simulink model "simLQR"  (R2015a)
settings: Solver=ode4  StartTime=0.0  StopTime=120  FixedStep=T  RelTol=1e-3
values from neighbouring files (symbols this model uses):
  aLeq = pnt(4)    [Data.m]
  aReq = pnt(3)    [Data.m]
  InitialValue = [0;0;0;rolleq;pitcheq;0;aReq;aLeq;0;0;0;0;0;0;0;0;reshape(AUX,256,1)]    [LinearAnalisys.m]
  pitcheq = pnt(2)    [Data.m]
  rolleq = pnt(1)    [Data.m]
  T = 12*(10^(-3))    (= 0.012)    [LinearAnalisys.m]
undefined symbols (not defined in the file or in its folder): K
settings Model: Creator=arthur  LastModifiedBy=macro
settings DebuggingCC: UnderspecifiedInitializationDetection=Classic  MergeDetectMultiDrivingBlocksExec=none  SolverPrmCheckMsg=warning  StateNameClashWarn=warning

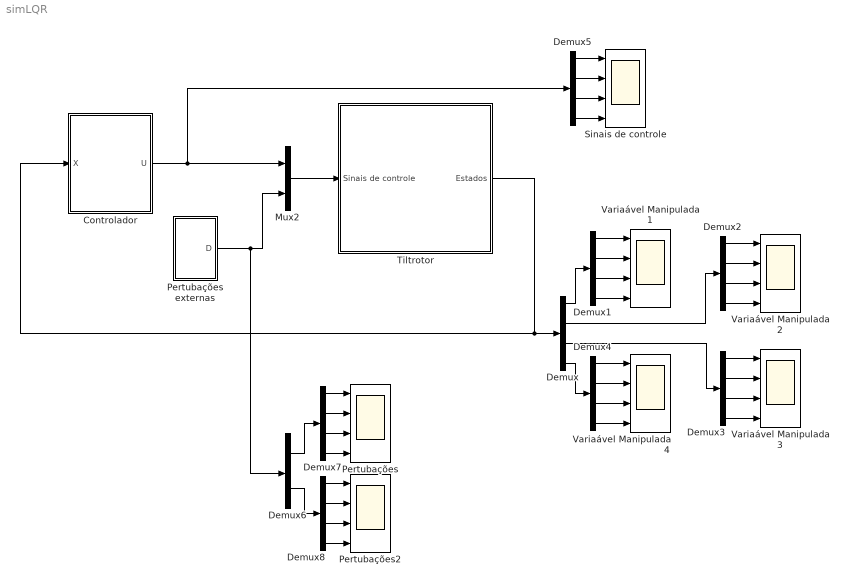
== system simLQR ==
  Controlador : Subsystem
      mask Display: image(imread('Photos/pc.jpg'))
  Demux{,1..5,7..8} (8 alike) : Demux
  Demux6 : Demux  Outputs=2
  Mux2 : Mux  Inputs=[4,8]
  Pertubações : Scope  NumInputPorts=4
      settings: YMin=-0.035~-0.5~-0.03~-0.3  YMax=0.005~3~0.005~0.05
  Pertubações externas : Subsystem
  Pertubações2 : Scope  NumInputPorts=4
      settings: YMin=-0.035~-0.5~-0.03~-0.3  YMax=0.005~3~0.005~0.05  SaveName=ScopeData2
  Sinais de controle : Scope  NumInputPorts=4
      settings: YMin=-0.035~-0.5~-0.03~-0.3  YMax=0.005~3~0.005~0.05
  Tiltrotor : Subsystem
      mask Display: image(imread('Photos/tilt.jpg'))
  Variaável Manipulada{1..4} (4 alike) : Scope  NumInputPorts=4
      Variaável Manipulada1 settings: YMin=-0.02~0.001~-0.08~0  YMax=0.05~0.009~-0.01~7  SaveName=ScopeData3
      Variaável Manipulada2 settings: YMin=-2~-55~-4250~-4000  YMax=2~-20~-2250~-2250  SaveName=ScopeData6
      Variaável Manipulada3 settings: YMin=-0.0045~-5~-5~-5  YMax=0.002~5~5~5  SaveName=ScopeData4
      Variaável Manipulada4 settings: YMin=0.055~-0.0195~-0.06475~-0.11  YMax=0.058~-0.0165~-0.06325~-0.055  SaveName=ScopeData5
  wires:
  Mux2/1 -> Tiltrotor/1(Sinais de controle)
  Pertubações externas/1(D) -> Demux6/1, Mux2/2
  Tiltrotor/1(Estados) -> Demux/1, Controlador/1(X)
  Demux/1 -> Demux1/1
  Demux1/1 -> Variaável Manipulada1/1
  Demux1/2 -> Variaável Manipulada1/2
  Demux1/3 -> Variaável Manipulada1/3
  Demux1/4 -> Variaável Manipulada1/4
  Demux/2 -> Demux2/1
  Demux2/1 -> Variaável Manipulada2/1
  Demux2/2 -> Variaável Manipulada2/2
  Demux2/3 -> Variaável Manipulada2/3
  Demux2/4 -> Variaável Manipulada2/4
  Demux/3 -> Demux3/1
  Demux3/1 -> Variaável Manipulada3/1
  Demux3/2 -> Variaável Manipulada3/2
  Demux3/3 -> Variaável Manipulada3/3
  Demux3/4 -> Variaável Manipulada3/4
  Demux/4 -> Demux4/1
  Demux4/1 -> Variaável Manipulada4/1
  Demux4/2 -> Variaável Manipulada4/2
  Demux4/3 -> Variaável Manipulada4/3
  Demux4/4 -> Variaável Manipulada4/4
  Demux5/1 -> Sinais de controle/1
  Demux5/2 -> Sinais de controle/2
  Demux5/3 -> Sinais de controle/3
  Demux5/4 -> Sinais de controle/4
  Demux6/1 -> Demux7/1
  Demux7/1 -> Pertubações/1
  Demux7/2 -> Pertubações/2
  Demux7/3 -> Pertubações/3
  Demux7/4 -> Pertubações/4
  Demux6/2 -> Demux8/1
  Demux8/1 -> Pertubações2/1
  Demux8/2 -> Pertubações2/2
  Demux8/3 -> Pertubações2/3
  Demux8/4 -> Pertubações2/4
  Controlador/1(U) -> Mux2/1, Demux5/1

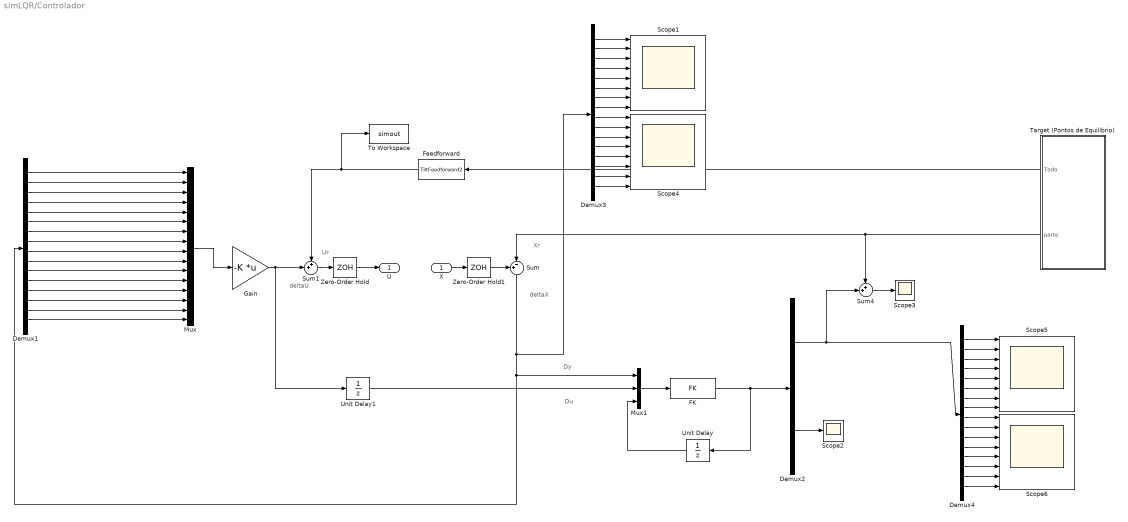
== system simLQR/Controlador ==
  note: Du
  note: Dy
  note: Xr
  note: deltaX
  note: Ur
  note: deltaU
  X : Inport
  Demux1 : Demux  Outputs=16
  Demux2 : Demux  Outputs=[16,256]
  Demux3 : Demux  Outputs=16
  Demux4 : Demux  Outputs=16
  FK : MATLABFcn  MATLABFcn=FK  OutputDimensions=272
  Feedforward : MATLABFcn  MATLABFcn=TiltFeedforward2  OutputDimensions=4
  Gain : Gain  Gain=-K  Multiplication=Matrix(K*u) (u vector)
  Mux : Mux  Inputs=16
  Mux1 : Mux  Inputs=[16,4,272]
  Scope{1,4..6} (4 alike) : Scope  NumInputPorts=8
      Scope1 settings: YMin=-0.0001~-0.000125~-0.00015~0.001925~0.052~0.0005~-0.05466~-0.05164  YMax=0.0009~2.5e-05~5e-05~0.002075~0.05375~0.0035~-0.05461~-0.05159  SaveName=ScopeData8
      Scope4 settings: YMin=-0.055~-5~-5~-5~-5~-5~-5~-5  YMax=0.055~5~5~5~5~5~5~5  SaveName=ScopeData11
      Scope5 settings: YMin=0.00075~7.5e-05~-9e-05~-0.00749~0.0434~0.00125~-0.04485~-0.042475  YMax=0.002~0.0002~1e-05~-0.00743~0.0439~0.003~-0.04477~-0.042375  SaveName=ScopeData7
      Scope6 settings: YMin=-0.055~-5~-5~-5~-5~-5~-5~-5  YMax=0.055~5~5~5~5~5~5~5  SaveName=ScopeData12
  Scope2 : Scope
      settings: YMin=-7e+09  YMax=7e+09  SaveName=ScopeData9
  Scope3 : Scope
      settings: YMin=-5e-06  YMax=5e-06  SaveName=ScopeData10
  Sum : Sum  Inputs=+-|
  Sum1 : Sum  Inputs=++|
  Sum4 : Sum  Inputs=++|
  Target (Pontos de Equilíbrio) : Subsystem
      mask Display: image(imread('Photos/alvo.jpg'))
  To Workspace : ToWorkspace  VariableName=simout  SampleTime=-1
  Unit Delay : UnitDelay  InitialCondition=InitialValue  SampleTime=T
  Unit Delay1 : UnitDelay  InitialCondition=[0,0,0,0]  SampleTime=T
  Zero-Order Hold : ZeroOrderHold  SampleTime=T
  Zero-Order Hold1 : ZeroOrderHold  SampleTime=T
  U : Outport
  wires:
  Feedforward/1 -> To Workspace/1, Sum1/1
  Demux1/5 -> Mux/5
  Demux1/15 -> Mux/15
  Demux1/14 -> Mux/14
  Demux1/11 -> Mux/11
  Demux1/13 -> Mux/13
  Demux1/12 -> Mux/12
  Demux1/1 -> Mux/1
  Mux/1 -> Gain/1
  Demux1/9 -> Mux/9
  Demux1/16 -> Mux/16
  Demux1/4 -> Mux/4
  Demux1/7 -> Mux/7
  Demux1/3 -> Mux/3
  Demux1/2 -> Mux/2
  Demux1/10 -> Mux/10
  Demux1/6 -> Mux/6
  Demux1/8 -> Mux/8
  Target (Pontos de Equilíbrio)/1(Todo) -> Feedforward/1
  Target (Pontos de Equilíbrio)/2(parte) -> Sum/2, Sum4/1
  Sum1/1 -> Zero-Order Hold/1
  X/1 -> Zero-Order Hold1/1
  Zero-Order Hold/1 -> U/1
  Zero-Order Hold1/1 -> Sum/1
  Mux1/1 -> FK/1
  FK/1 -> Demux2/1, Unit Delay/1
  Sum/1 -> Demux3/1, Demux1/1, Mux1/1
  Gain/1 -> Unit Delay1/1, Sum1/2
  Demux2/2 -> Scope2/1
  Unit Delay1/1 -> Mux1/2
  Sum4/1 -> Scope3/1
  Demux3/1 -> Scope1/1
  Demux3/8 -> Scope1/8
  Demux3/7 -> Scope1/7
  Demux3/6 -> Scope1/6
  Demux3/5 -> Scope1/5
  Demux3/4 -> Scope1/4
  Demux3/3 -> Scope1/3
  Demux3/2 -> Scope1/2
  Demux3/16 -> Scope4/8
  Demux3/15 -> Scope4/7
  Demux3/14 -> Scope4/6
  Demux3/12 -> Scope4/4
  Demux3/13 -> Scope4/5
  Demux3/11 -> Scope4/3
  Demux3/10 -> Scope4/2
  Demux3/9 -> Scope4/1
  Demux2/1 -> Demux4/1, Sum4/2
  Demux4/8 -> Scope5/8
  Demux4/7 -> Scope5/7
  Demux4/6 -> Scope5/6
  Demux4/5 -> Scope5/5
  Demux4/4 -> Scope5/4
  Demux4/3 -> Scope5/3
  Demux4/2 -> Scope5/2
  Demux4/12 -> Scope6/4
  Demux4/11 -> Scope6/3
  Demux4/10 -> Scope6/2
  Demux4/9 -> Scope6/1
  Demux4/1 -> Scope5/1
  Demux4/13 -> Scope6/5
  Demux4/14 -> Scope6/6
  Demux4/15 -> Scope6/7
  Demux4/16 -> Scope6/8
  Unit Delay/1 -> Mux1/3

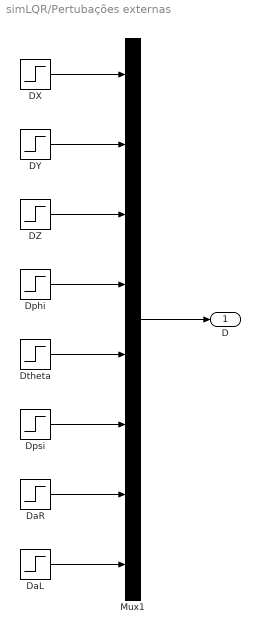
== system simLQR/Pertubações externas ==
  DX : Step  After=0  SampleTime=0
  DY : Step  After=0  SampleTime=0
  DZ : Step  After=0  SampleTime=0
  DaL : Step  After=0  SampleTime=0
  DaR : Step  After=0  SampleTime=0
  Dphi : Step  After=0  SampleTime=0
  Dpsi : Step  After=0  SampleTime=0
  Dtheta : Step  After=0  SampleTime=0
  Mux1 : Mux  Inputs=8
  D : Outport
  wires:
  Dphi/1 -> Mux1/4
  DaL/1 -> Mux1/8
  DaR/1 -> Mux1/7
  Dpsi/1 -> Mux1/6
  Dtheta/1 -> Mux1/5
  Mux1/1 -> D/1
  DZ/1 -> Mux1/3
  DY/1 -> Mux1/2
  DX/1 -> Mux1/1

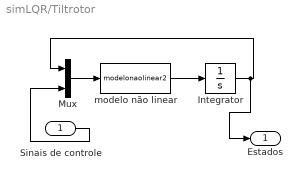
== system simLQR/Tiltrotor ==
  Sinais de controle : Inport
  Integrator : Integrator  InitialCondition=[0,0,0,rolleq,pitcheq,0,aReq,aLeq,0,0,0,0,0,0,0,0]
  Mux : Mux  Inputs=2
  modelo não linear : MATLABFcn  MATLABFcn=modelonaolinear2  OutputDimensions=16
  Estados : Outport
  wires:
  Mux/1 -> modelo não linear/1
  modelo não linear/1 -> Integrator/1
  Sinais de controle/1 -> Mux/2
  Integrator/1 -> Mux/1, Estados/1

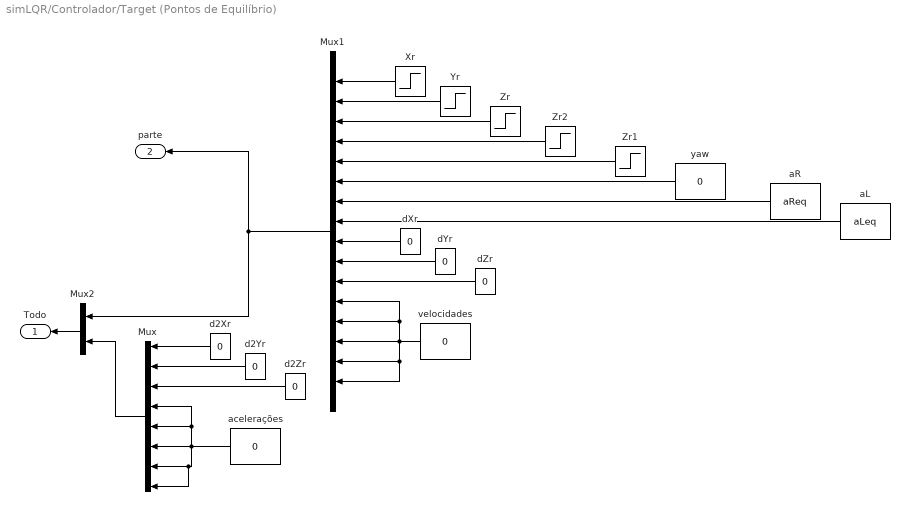
== system simLQR/Controlador/Target (Pontos de Equilíbrio) ==
  Mux : Mux  Inputs=8
  Mux1 : Mux  Inputs=16
  Mux2 : Mux  Inputs=2
  Xr : Step  Time=0  After=0  SampleTime=0
  Yr : Step  Time=0  After=0  SampleTime=0
  Zr : Step  Before=0.001  After=0  SampleTime=0
  Zr1 : Step  Time=0  Before=pitcheq  After=pitcheq  SampleTime=0
  Zr2 : Step  Time=0  Before=rolleq  After=rolleq  SampleTime=0
  aL : Constant  Value=aLeq
  aR : Constant  Value=aReq
  acelerações : Constant  Value=0
  d2Xr : Constant  Value=0
  d2Yr : Constant  Value=0
  d2Zr : Constant  Value=0
  dXr : Constant  Value=0
  dYr : Constant  Value=0
  dZr : Constant  Value=0
  velocidades : Constant  Value=0
  yaw : Constant  Value=0
  Todo : Outport
  parte : Outport  Port=2
  wires:
  Yr/1 -> Mux1/2
  Zr/1 -> Mux1/3
  Mux1/1 -> Mux2/1, parte/1
  Xr/1 -> Mux1/1
  Zr2/1 -> Mux1/4
  yaw/1 -> Mux1/6
  aR/1 -> Mux1/7
  aL/1 -> Mux1/8
  velocidades/1 -> Mux1/13, Mux1/12, Mux1/16, Mux1/15, Mux1/14
  dXr/1 -> Mux1/9
  dYr/1 -> Mux1/10
  dZr/1 -> Mux1/11
  d2Xr/1 -> Mux/1
  d2Yr/1 -> Mux/2
  d2Zr/1 -> Mux/3
  Mux2/1 -> Todo/1
  Mux/1 -> Mux2/2
  acelerações/1 -> Mux/8, Mux/7, Mux/6, Mux/5, Mux/4
  Zr1/1 -> Mux1/5
